simulink model "session_practice"  (R2020a)
settings: Solver=VariableStepAuto  StartTime=0.0  StopTime=10.0  RelTol=1e-3
settings Model: Creator=Ganesh  LastModifiedBy=Ganesh

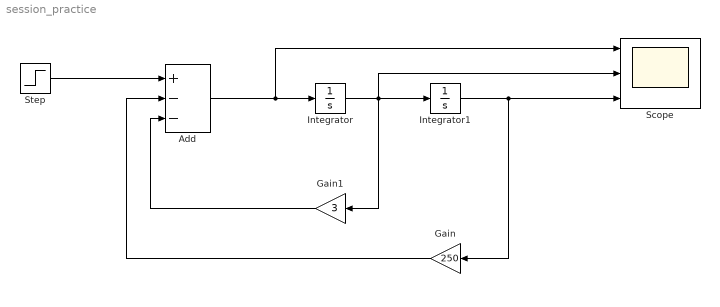
== system session_practice ==
  Add : Sum  Inputs=+--
  Gain : Gain  Gain=250
  Gain1 : Gain  Gain=3
  Integrator : Integrator
  Integrator1 : Integrator
  Scope : Scope  NumInputPorts=3
  Step : Step  Time=0  After=5  SampleTime=0
  wires:
  Add/1 -> Scope/1, Integrator/1
  Integrator/1 -> Gain1/1, Scope/2, Integrator1/1
  Integrator1/1 -> Gain/1, Scope/3
  Gain1/1 -> Add/3
  Gain/1 -> Add/2
  Step/1 -> Add/1
